simulink model "Reaction_model"  (R2020b)
settings: Solver=FixedStepAuto  StartTime=0.0  StopTime=1178520  FixedStep=10  RelTol=1e-5
settings Model: OrderedModelArguments=off  Creator=20181234  LastModifiedBy=20181234
settings SolverCC: ConcurrentTasks=on  AutoInsertRateTranBlk=on

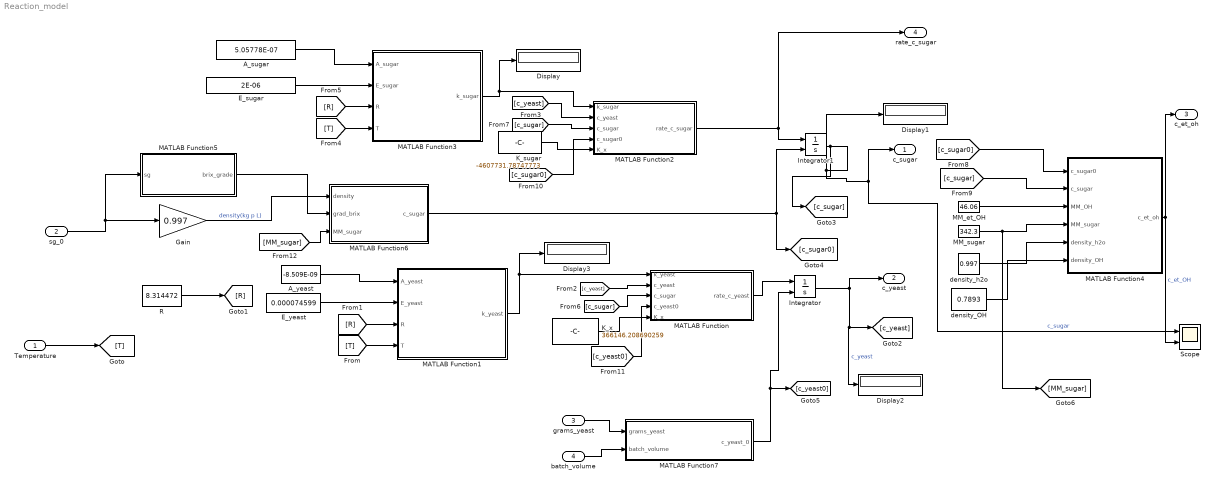
== system Reaction_model ==
  Temperature : Inport
  sg_0 : Inport  Port=2
  grams_yeast : Inport  Port=3
  batch_volume : Inport  Port=4
  A_sugar : Constant  Value=5.05778E-07
  A_yeast : Constant  Value=-8.509E-09
  Display{,1..3} (4 alike) : Display
  E_sugar : Constant  Value=2E-06
  E_yeast : Constant  Value=0.000074599
  Gain : Gain  Gain=0.997
  Integrator : Integrator  InitialConditionSource=external
  Integrator1 : Integrator  InitialConditionSource=external
  K_sugar : Constant  Value=-4607731.78747773
  K_x : Constant  Value=366146.208690259
  MATLAB Function : MATLAB Function  TreatAsAtomicUnit=on
  MATLAB Function1 : MATLAB Function  TreatAsAtomicUnit=on
  MATLAB Function2 : MATLAB Function  TreatAsAtomicUnit=on
  MATLAB Function3 : MATLAB Function  TreatAsAtomicUnit=on
  MATLAB Function4 : MATLAB Function  TreatAsAtomicUnit=on
  MATLAB Function5 : MATLAB Function  TreatAsAtomicUnit=on
  MATLAB Function6 : MATLAB Function  TreatAsAtomicUnit=on
  MATLAB Function7 : MATLAB Function  TreatAsAtomicUnit=on
  MM_et_OH : Constant  Value=46.06
  MM_sugar : Constant  Value=342.3
  R : Constant  Value=8.314472
  Scope : Scope  NumInputPorts=2
  density_OH : Constant  Value=0.7893
  density_h2o : Constant  Value=0.997
  c_sugar : Outport
  c_yeast : Outport  Port=2
  c_et_oh : Outport  Port=3
  rate_c_sugar : Outport  Port=4
  wires:
  Integrator/1 -> Display2/1, [c_yeast], c_yeast/1  "c_yeast"
  MATLAB Function/1(rate_c_yeast) -> Integrator/1
  MATLAB Function1/1(k_yeast) -> Display3/1, MATLAB Function/1(k_yeast)
  R/1 -> [R]
  [T] -> MATLAB Function1/4(T)
  [R] -> MATLAB Function1/3(R)
  A_yeast/1 -> MATLAB Function1/1(A_yeast)
  E_yeast/1 -> MATLAB Function1/2(E_yeast)
  Integrator1/1 -> [c_sugar], Scope/1, c_sugar/1, Display1/1  "c_sugar"
  [c_yeast] -> MATLAB Function/2(c_yeast)
  MATLAB Function2/1(rate_c_sugar) -> Integrator1/1, rate_c_sugar/1
  [c_yeast] -> MATLAB Function2/2(c_yeast)
  MATLAB Function3/1(k_sugar) -> MATLAB Function2/1(k_sugar), Display/1
  [T] -> MATLAB Function3/4(T)
  [R] -> MATLAB Function3/3(R)
  E_sugar/1 -> MATLAB Function3/2(E_sugar)
  A_sugar/1 -> MATLAB Function3/1(A_sugar)
  K_x/1 -> MATLAB Function/5(K_x)
  K_sugar/1 -> MATLAB Function2/5(K_x)
  [c_sugar] -> MATLAB Function/3(c_sugar)
  [c_sugar] -> MATLAB Function2/3(c_sugar)
  [c_sugar0] -> MATLAB Function4/1(c_sugar0)
  [c_sugar] -> MATLAB Function4/2(c_sugar)
  MM_sugar/1 -> [MM_sugar], MATLAB Function4/4(MM_sugar)
  MM_et_OH/1 -> MATLAB Function4/3(MM_OH)
  MATLAB Function4/1(c_et_oh) -> c_et_oh/1, Scope/2  "c_et_OH"
  density_h2o/1 -> MATLAB Function4/5(density_h2o)
  density_OH/1 -> MATLAB Function4/6(density_OH)
  [c_sugar0] -> MATLAB Function2/4(c_sugar0)
  [c_yeast0] -> MATLAB Function/4(c_yeast0)
  MATLAB Function6/1(c_sugar) -> Integrator1/2, [c_sugar0]
  MATLAB Function7/1(c_yeast_0) -> Integrator/2, [c_yeast0]
  Temperature/1 -> [T]
  sg_0/1 -> MATLAB Function5/1(sg), Gain/1
  Gain/1 -> MATLAB Function6/1(density)  "density(kg p L)"
  MATLAB Function5/1(brix_grade) -> MATLAB Function6/2(grad_brix)
  [MM_sugar] -> MATLAB Function6/3(MM_sugar)
  grams_yeast/1 -> MATLAB Function7/1(grams_yeast)
  batch_volume/1 -> MATLAB Function7/2(batch_volume)

== matlab function Reaction_model/MATLAB Function1 ==
  data: A_yeast input; k_yeast output; E_yeast input; R input; T input
function k_yeast = fcn_k_yeast(A_yeast,E_yeast,R,T)

   k_yeast = A_yeast*exp(-E_yeast/(R*T));

== matlab function Reaction_model/MATLAB Function ==
  data: k_yeast input; rate_c_yeast output; c_yeast input; c_sugar input; c_yeast0 input; K_x input
function rate_c_yeast = fcn_R_yeast(k_yeast,c_yeast,c_sugar,c_yeast0,K_x)

    rate_c_yeast = k_yeast*c_yeast*c_sugar*K_x/(K_x+(-c_yeast0+c_yeast)^2);

== matlab function Reaction_model/MATLAB Function2 ==
  data: k_sugar input; rate_c_sugar output; c_yeast input; c_sugar input; c_sugar0 input; K_x input
function rate_c_sugar = fcn_R_sugar( k_sugar,c_yeast,c_sugar,c_sugar0,K_x)

    %rate_c_sugar = -k_sugar*c_yeast*c_sugar*K_x/(K_x+(-c_yeast0+c_yeast));
    rate_c_sugar = -k_sugar*c_yeast*c_sugar*K_x/(K_x+(c_sugar0-c_sugar)^2);

== matlab function Reaction_model/MATLAB Function3 ==
  data: A_sugar input; k_sugar output; E_sugar input; R input; T input
function k_sugar = fcn_k_sugar(A_sugar,E_sugar,R,T)

   k_sugar = A_sugar*exp(-E_sugar/(R*T));

== matlab function Reaction_model/MATLAB Function4 ==
  data: c_sugar0 input; c_et_oh output; c_sugar input; MM_OH input; MM_sugar input; density_h2o input; density_OH input
function c_et_oh = fc_et_oh(c_sugar0,c_sugar,MM_OH,MM_sugar,density_h2o, density_OH)

    c_et_oh = (c_sugar0-c_sugar)*MM_sugar/MM_OH*(density_OH/density_h2o)*(51.31533/100);

== matlab function Reaction_model/MATLAB Function5 ==
  data: sg input; brix_grade output
function brix_grade = fbrix(sg)

brix_grade = 143.254*(sg)^3-648.67*(sg)^2+1125.805*(sg)-620.389;

== matlab function Reaction_model/MATLAB Function6 ==
  data: density input; c_sugar output; grad_brix input; MM_sugar input
function c_sugar = fc_sugar(density,grad_brix,MM_sugar)

c_sugar=density*grad_brix*10/MM_sugar*1000;

== matlab function Reaction_model/MATLAB Function7 ==
  data: grams_yeast input; c_yeast_0 output; batch_volume input
function c_yeast_0 = fc_yeast_0(grams_yeast,batch_volume)
MM_yeast=180.1559;
c_yeast_0 = (grams_yeast/batch_volume)/MM_yeast*1000;
